simulink model "cl3"  (R2019b)
settings: Solver=VariableStepAuto  StartTime=0.0  StopTime=10.0  RelTol=1e-3
values from neighbouring files (symbols this model uses):
  A = [[0 0 1 0] ... (first row only)    [ClosedLoop.m]    (also in Inverted_pendulum.m; Realistic_model.m)
  B = [0 ... (first row only)    [ClosedLoop.m]    (also in Inverted_pendulum.m; Realistic_model.m)
  C = eye(n)    [ClosedLoop.m]    (also in Inverted_pendulum.m = [4.41/0.456, 0, 0, 0; Realistic_model.m = zeros(n,n); C(1,1) = 1; C(2,2) = 1)
  C_cl = C    [ClosedLoop.m]    (also in Realistic_model.m = C-D*K)
  D = zeros(n,1)    [ClosedLoop.m]    (also in Inverted_pendulum.m = [0;0]; Realistic_model.m)
  Nu = N(5,:)    [ClosedLoop.m]
  Nx = N(1:4,:)    [ClosedLoop.m]
undefined symbols (not defined in the file or in its folder): K
settings Model: Creator=elina  LastModifiedBy=elina

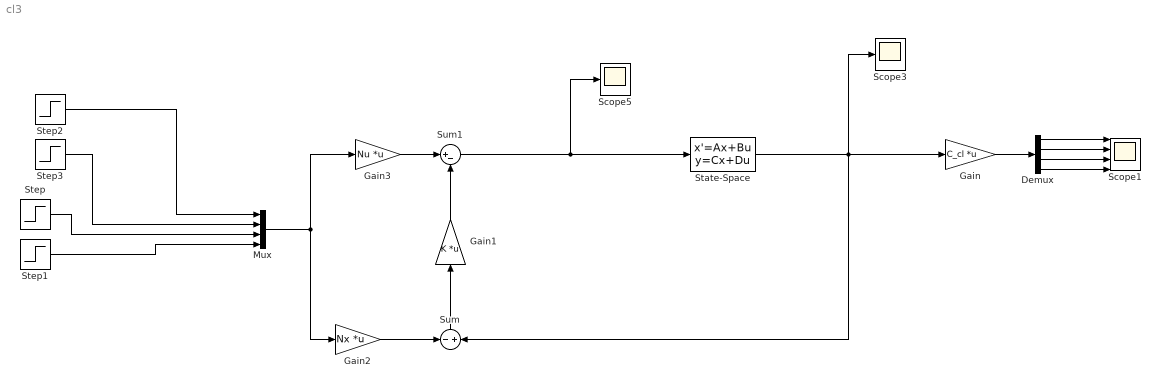
== system cl3 ==
  Demux : Demux
  Gain : Gain  Gain=C_cl  Multiplication=Matrix(K*u)
  Gain1 : Gain  Gain=K  Multiplication=Matrix(K*u)
  Gain2 : Gain  Gain=Nx  Multiplication=Matrix(K*u)
  Gain3 : Gain  Gain=Nu  Multiplication=Matrix(K*u)
  Mux : Mux
  Scope1 : Scope  NumInputPorts=4
  Scope3 : Scope
  Scope5 : Scope
  State-Space : StateSpace  A=A  B=B  C=C  D=D  InitialCondition=0
  Step : Step  Time=0  After=0  SampleTime=0
  Step1 : Step  Time=0  After=0  SampleTime=0
  Step2 : Step  Time=0  After=2  SampleTime=0
  Step3 : Step  After=0  SampleTime=0
  Sum : Sum  Inputs=-|+
  Sum1 : Sum  Inputs=|+-
  wires:
  Gain/1 -> Demux/1
  Demux/1 -> Scope1/1
  Demux/2 -> Scope1/2
  Demux/3 -> Scope1/3
  Demux/4 -> Scope1/4
  State-Space/1 -> Sum/2, Scope3/1, Gain/1
  Step3/1 -> Mux/2
  Step/1 -> Mux/3
  Step1/1 -> Mux/4
  Gain2/1 -> Sum/1
  Sum/1 -> Gain1/1
  Gain3/1 -> Sum1/1
  Gain1/1 -> Sum1/2
  Sum1/1 -> Scope5/1, State-Space/1
  Step2/1 -> Mux/1
  Mux/1 -> Gain2/1, Gain3/1
